simulink model "ROPOD_4Wheel_Tdistkinb_cntr_modular_Code_GEN"  (R2020b)
settings: Solver=VariableStepAuto  StartTime=0.0  StopTime=10.0  RelTol=1e-3
values from neighbouring files (symbols this model uses):
  FFtheta_intia = 0    [init_model.m]
  FFxy_mass = 0*80    (= 0)    [init_model.m]
  I_fhz_dtheta_cntr = 0.3    [init_model.m]
  I_fhz_dvarphi_cntr = 0    [init_model.m]
  I_fhz_dxdy_cntr = 0.25    [init_model.m]
  K_gain_dtheta_cntr = 150    [init_model.m]
  K_gain_dvarphi_cntr = 0.05    [init_model.m]
  K_gain_dxdy_cntr = 200    [init_model.m]
  LL_wp_fhz_dtheta_cntr = 20    [init_model.m]
  LL_wp_fhz_dvarphi_cntr = 10    [init_model.m]
  LL_wp_fhz_dxdy_cntr = 20    [init_model.m]
  LL_wz_fhz_dtheta_cntr = 20    [init_model.m]
  LL_wz_fhz_dvarphi_cntr = 2    [init_model.m]
  LL_wz_fhz_dxdy_cntr = 20    [init_model.m]
  LPF_fhz_ddelta_meas = 50    [init_model.m]
  LPF_fhz_dtheta_cntr = 100    [init_model.m]
  LPF_fhz_dvarphi_cntr = 50    [init_model.m]
  LPF_fhz_dvarphi_meas = 50    [init_model.m]
  LPF_fhz_dxdy_cntr = 100    [init_model.m]
  max_hw_tau = 7.0    (= 7)    [init_model.m]
  max_ropod_acc_theta = 1.6    [init_model.m]
  max_ropod_acc_xy = 2.0    (= 2)    [init_model.m]
  max_ropod_sw_force = 500    [init_model.m]
  max_ropod_sw_tau = 250    [init_model.m]
  max_ropod_vel_theta = 1.6    [init_model.m]
  max_ropod_vel_xy = 2.0    (= 2)    [init_model.m]
  max_sw_current = 10    [init_model.m]
  Nwheels = 4    [Jqwl_numeric_function.m]    (also in S_matrix.m; extract_kinmodel_parameters.m; init_model.m; tau_optimal_dist_vec_fun.m)
  pivot_offs_sws = [0.0243    0.4689    0.3384    5.9050]    [init_model.m]
  ropod_kinmodel_pv = struct2array(ropod_kinmodel_param)    [set_ropod_KinModparams.m]
  SW_COM1_ENABLE1 = hex2dec('0001')    [init_model.m]
  SW_COM1_ENABLE2 = hex2dec('0002')    [init_model.m]
  SW_COM1_MODE_TORQUE = bitshift(hex2dec('0000'),2)    [init_model.m]
  SW_COM1_MODE_VELOCITY = bitshift(hex2dec('0002'),2)    [init_model.m]
  SW_COM1_USE_TS = hex2dec('8000')    [init_model.m]
  sw_tau_2_current = 1/motor_physical_parameters.torqueconstant.value    [init_model.m]
  Tinit = 2    [init_model.m]
  Ts = 0.001    [init_model.m]
undefined symbols (not defined in the file or in its folder): DiscIntNeverNeededParam
libraries: simulink x25, cstblocks x23, pid_lib x22, dspsigops x12, SOEM_EtherCAT_Lib x5
(part 1 of 4)
settings Model: Creator=cesar  LastModifiedBy=cesar
settings DataIOCC: ReturnWorkspaceOutputs=off
settings OptimizationCC: DefaultParameterBehavior=Inlined  UseFloatMulNetSlope=on  InlineInvariantSignals=on  EfficientFloat2IntCast=on
settings DebuggingCC: UnderSpecifiedDataTypeMsg=warning  ArithmeticOperatorsInVariantConditions=warning
settings HardwareCC: ProdBitPerLong=64  ProdHWDeviceType=Intel->x86-64 (Linux 64)
settings SFSimCC: SimUseLocalCustomCode=off  CustomCodeUndefinedFunction=UseInterfaceOnly
settings RTWCC: GenCodeOnly=on  RTWUseLocalCustomCode=off  BuildConfiguration=Faster Runs
settings GRTTargetCC: MatFileLogging=off  SupportNonFinite=off

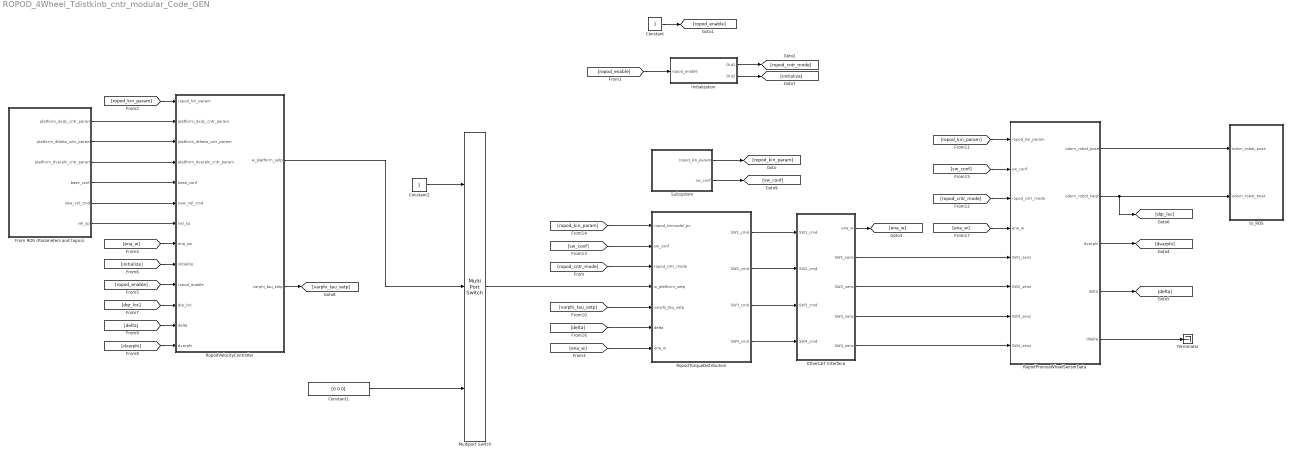
== system ROPOD_4Wheel_Tdistkinb_cntr_modular_Code_GEN ==
  Constant : Constant
  Constant1 : Constant  Value=[0 0 0]
  Constant2 : Constant
  EtherCAT Interface : Subsystem
  From ROS (Parameters and topics) : Subsystem
  Initialization : Subsystem
  Multiport Switch : MultiPortSwitch  Inputs=2
  RopodProcessWheelSensorData : Subsystem
  RopodTorqueDistribution : Subsystem
  RopodVelocityController : Subsystem
  Subsystem : Subsystem
  Terminator : Terminator
  to_ROS : Subsystem
  wires:
  RopodProcessWheelSensorData/1(odom_robot_pose) -> to_ROS/1(odom_robot_pose)
  RopodProcessWheelSensorData/2(odom_robot_twist) -> [dqr_loc], to_ROS/2(odom_robot_twist)
  RopodTorqueDistribution/4(SW4_cmd) -> EtherCAT Interface/4(SW4_cmd)
  RopodTorqueDistribution/3(SW3_cmd) -> EtherCAT Interface/3(SW3_cmd)
  RopodTorqueDistribution/2(SW2_cmd) -> EtherCAT Interface/2(SW2_cmd)
  RopodTorqueDistribution/1(SW1_cmd) -> EtherCAT Interface/1(SW1_cmd)
  From ROS (Parameters and topics)/1(platform_dxdy_cntr_param) -> RopodVelocityController/2(platform_dxdy_cntr_param)
  From ROS (Parameters and topics)/2(platform_dtheta_cntr_param) -> RopodVelocityController/3(platform_dtheta_cntr_param)
  From ROS (Parameters and topics)/3(platform_dvarphi_cntr_param) -> RopodVelocityController/4(platform_dvarphi_cntr_param)
  From ROS (Parameters and topics)/4(base_conf) -> RopodVelocityController/5(base_conf)
  From ROS (Parameters and topics)/5(new_vel_cmd) -> RopodVelocityController/6(new_vel_cmd)
  From ROS (Parameters and topics)/6(vel_sp) -> RopodVelocityController/7(vel_sp)
  [ropod_cntr_mode] -> RopodTorqueDistribution/3(ropod_cntr_mode)
  [ropod_enable] -> Initialization/1(ropod_enable)
  Initialization/1(Out1) -> [ropod_cntr_mode]
  Initialization/2(Out2) -> [initialize]
  Constant/1 -> [ropod_enable]
  [ropod_kin_param] -> RopodVelocityController/1(ropod_kin_param)
  [ena_w] -> RopodTorqueDistribution/7(ena_w)
  [ena_w] -> RopodVelocityController/8(ena_sw)
  [ropod_enable] -> RopodVelocityController/10(ropod_enable)
  [initialize] -> RopodVelocityController/9(initialize)
  RopodProcessWheelSensorData/3(dvarphi) -> [dvarphi]
  RopodProcessWheelSensorData/4(delta) -> [delta]
  RopodProcessWheelSensorData/5(ddelta) -> Terminator/1
  [dqr_loc] -> RopodVelocityController/11(dqr_loc)
  [dvarphi] -> RopodVelocityController/13(dvarphi)
  [delta] -> RopodVelocityController/12(delta)
  RopodVelocityController/2(varphi_tau_setp) -> [varphi_tau_setp]
  [varphi_tau_setp] -> RopodTorqueDistribution/5(varphi_tau_setp)
  Constant2/1 -> Multiport Switch/1
  Constant1/1 -> Multiport Switch/3
  RopodVelocityController/1(w_platform_setp) -> Multiport Switch/2
  [ropod_kin_param] -> RopodProcessWheelSensorData/1(ropod_kin_param)
  [ropod_cntr_mode] -> RopodProcessWheelSensorData/3(ropod_cntr_mode)
  Subsystem/1(ropod_kin_param) -> [ropod_kin_param]
  Subsystem/2(sw_conf) -> [sw_conf]
  [sw_conf] -> RopodTorqueDistribution/2(sw_conf)
  [ropod_kin_param] -> RopodTorqueDistribution/1(ropod_kinmodel_pv)
  [sw_conf] -> RopodProcessWheelSensorData/2(sw_conf)
  EtherCAT Interface/1(ena_w) -> [ena_w]
  EtherCAT Interface/2(SW1_sens) -> RopodProcessWheelSensorData/5(SW1_sens)
  EtherCAT Interface/3(SW2_sens) -> RopodProcessWheelSensorData/6(SW2_sens)
  EtherCAT Interface/4(SW3_sens) -> RopodProcessWheelSensorData/7(SW3_sens)
  EtherCAT Interface/5(SW4_sens) -> RopodProcessWheelSensorData/8(SW4_sens)
  [delta] -> RopodTorqueDistribution/6(delta)
  Multiport Switch/1 -> RopodTorqueDistribution/4(w_platform_setp)
  [ena_w] -> RopodProcessWheelSensorData/4(ena_w)

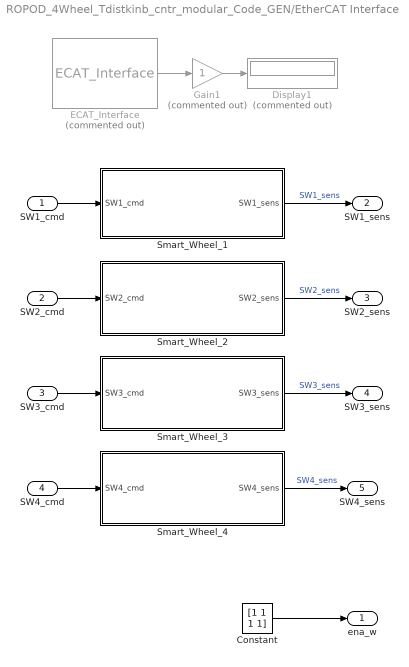
== system ROPOD_4Wheel_Tdistkinb_cntr_modular_Code_GEN/EtherCAT Interface ==
  SW1_cmd : Inport
  SW2_cmd : Inport  Port=2
  SW3_cmd : Inport  Port=3
  SW4_cmd : Inport  Port=4
  Constant : Constant  Value=[1 1 1 1]
  Display1 : Display  Commented=on
  ECAT_Interface : SOEM_EtherCAT_Lib/ECAT_Interface  Priority=0  Commented=on  IFINTERFACE=eth0  TS=Ts
      settings: SourceProductName=SOEM_EtherCAT_Lib
  Gain1 : Gain  Commented=on  OutDataTypeStr=double
  Smart_Wheel_1 : Subsystem
  Smart_Wheel_2 : Subsystem
  Smart_Wheel_3 : Subsystem
  Smart_Wheel_4 : Subsystem
  ena_w : Outport  VectorParamsAs1DForOutWhenUnconnected=off
  SW1_sens : Outport  Port=2  VectorParamsAs1DForOutWhenUnconnected=off
  SW2_sens : Outport  Port=3  VectorParamsAs1DForOutWhenUnconnected=off
  SW3_sens : Outport  Port=4  VectorParamsAs1DForOutWhenUnconnected=off
  SW4_sens : Outport  Port=5  VectorParamsAs1DForOutWhenUnconnected=off
  wires:
  Smart_Wheel_2/1(SW2_sens) -> SW2_sens/1  "SW2_sens"
  Smart_Wheel_3/1(SW3_sens) -> SW3_sens/1  "SW3_sens"
  SW4_cmd/1 -> Smart_Wheel_4/1(SW4_cmd)
  SW2_cmd/1 -> Smart_Wheel_2/1(SW2_cmd)
  SW3_cmd/1 -> Smart_Wheel_3/1(SW3_cmd)
  SW1_cmd/1 -> Smart_Wheel_1/1(SW1_cmd)
  Smart_Wheel_1/1(SW1_sens) -> SW1_sens/1  "SW1_sens"
  Smart_Wheel_4/1(SW4_sens) -> SW4_sens/1  "SW4_sens"
  ECAT_Interface/1 -> Gain1/1
  Gain1/1 -> Display1/1
  Constant/1 -> ena_w/1

== system ROPOD_4Wheel_Tdistkinb_cntr_modular_Code_GEN/From ROS (Parameters and topics) ==
  note: doing the transformation with the angle from odometry data helps
      | to keep the robot better align during the Identification, especially because
      | we do not have any absolute reference
  Constant1 : Constant
  Controllers conf : Subsystem
  From Workspace1 : FromWorkspace  VariableName=qrefdot
  Gain1 : Gain
  ROS base conf : Subsystem
  Selector1 : Selector  InputPortWidth=3  IndexOptions=Index vector (dialog)  Indices=3  OutputSizes=1
  rot_matrix2 : MATLAB Function  TreatAsAtomicUnit=on
  platform_dxdy_cntr_param : Outport  VectorParamsAs1DForOutWhenUnconnected=off
  platform_dtheta_cntr_param : Outport  Port=2  VectorParamsAs1DForOutWhenUnconnected=off
  platform_dvarphi_cntr_param : Outport  Port=3  VectorParamsAs1DForOutWhenUnconnected=off
  base_conf : Outport  Port=4  VectorParamsAs1DForOutWhenUnconnected=off
  new_vel_cmd : Outport  Port=5  VectorParamsAs1DForOutWhenUnconnected=off
  vel_sp : Outport  Port=6  VectorParamsAs1DForOutWhenUnconnected=off
  wires:
  Controllers conf/1(platform_dxdy_cntr_param) -> platform_dxdy_cntr_param/1
  Constant1/1 -> new_vel_cmd/1
  Gain1/1 -> vel_sp/1
  ROS base conf/1(base_conf) -> base_conf/1
  From Workspace1/1 -> Selector1/1, rot_matrix2/1(dqr_glb)
  Controllers conf/3(platform_dvarphi_cntr_param) -> platform_dvarphi_cntr_param/1
  Controllers conf/2(platform_dtheta_cntr_param) -> platform_dtheta_cntr_param/1
  Selector1/1 -> rot_matrix2/2(theta)
  rot_matrix2/1(dqr_loc) -> Gain1/1

== system ROPOD_4Wheel_Tdistkinb_cntr_modular_Code_GEN/Initialization ==
  ropod_enable : Inport
  Allow Tinit seconds for initialization : simulink/Logic and Bit Operations/Compare To Constant  relop=<  const=Tinit  OutDataTypeStr=boolean
  Constant : Constant  Value=2
  Constant1 : Constant
  Constant2 : Constant  Value=0
  Digital Clock : DigitalClock  SampleTime=Ts
  Gain : Gain
  Gain1 : Gain  OutDataTypeStr=double
  Switch : Switch  Criteria=u2 > Threshold
  Switch1 : Switch  Criteria=u2 > Threshold
  Out1 : Outport  VectorParamsAs1DForOutWhenUnconnected=off
  Out2 : Outport  Port=2  VectorParamsAs1DForOutWhenUnconnected=off
  wires:
  Switch/1 -> Switch1/1
  Constant1/1 -> Switch/3
  Switch1/1 -> Gain/1
  Digital Clock/1 -> Allow Tinit seconds for initialization/1
  Allow Tinit seconds for initialization/1 -> Gain1/1, Switch/2
  Constant2/1 -> Switch1/3
  Constant/1 -> Switch/1
  ropod_enable/1 -> Switch1/2
  Gain/1 -> Out1/1
  Gain1/1 -> Out2/1

== system ROPOD_4Wheel_Tdistkinb_cntr_modular_Code_GEN/RopodProcessWheelSensorData ==
  ropod_kin_param : Inport
  sw_conf : Inport  Port=2
  ropod_cntr_mode : Inport  Port=3
  ena_w : Inport  Port=4
  SW1_sens : Inport  Port=5
  SW2_sens : Inport  Port=6
  SW3_sens : Inport  Port=7
  SW4_sens : Inport  Port=8
  Compare To Constant : simulink/Logic and Bit Operations/Compare To Constant  relop=~=  const=1  OutDataTypeStr=boolean
  Odometry and Measurement model 4SW : Subsystem
  ROPOD_4Wheel_sens : Subsystem
  odom_robot_pose : Outport  VectorParamsAs1DForOutWhenUnconnected=off
  odom_robot_twist : Outport  Port=2  VectorParamsAs1DForOutWhenUnconnected=off
  dvarphi : Outport  Port=3  VectorParamsAs1DForOutWhenUnconnected=off
  delta : Outport  Port=4  VectorParamsAs1DForOutWhenUnconnected=off
  ddelta : Outport  Port=5  VectorParamsAs1DForOutWhenUnconnected=off
  wires:
  ropod_kin_param/1 -> Odometry and Measurement model 4SW/1(param_in)
  Odometry and Measurement model 4SW/2(odom_robot_twist) -> odom_robot_twist/1
  SW2_sens/1 -> ROPOD_4Wheel_sens/4(SW2_sens)
  ROPOD_4Wheel_sens/3(ddelta) -> ddelta/1
  Odometry and Measurement model 4SW/1(odom_robot_pose) -> odom_robot_pose/1
  ROPOD_4Wheel_sens/2(delta) -> Odometry and Measurement model 4SW/4(delta), delta/1
  SW4_sens/1 -> ROPOD_4Wheel_sens/6(SW4_sens)
  ROPOD_4Wheel_sens/1(dvarphi) -> Odometry and Measurement model 4SW/3(dvarphi), dvarphi/1
  SW3_sens/1 -> ROPOD_4Wheel_sens/5(SW3_sens)
  SW1_sens/1 -> ROPOD_4Wheel_sens/3(SW1_sens)
  Compare To Constant/1 -> ROPOD_4Wheel_sens/1(disable)
  sw_conf/1 -> ROPOD_4Wheel_sens/2(sw_conf)
  ropod_cntr_mode/1 -> Compare To Constant/1
  ena_w/1 -> Odometry and Measurement model 4SW/2(ena_w)

== system ROPOD_4Wheel_Tdistkinb_cntr_modular_Code_GEN/RopodTorqueDistribution ==
  ropod_kinmodel_pv : Inport
  sw_conf : Inport  Port=2
  ropod_cntr_mode : Inport  Port=3
  w_platform_setp : Inport  Port=4
  varphi_tau_setp : Inport  Port=5
  delta : Inport  Port=6
  ena_w : Inport  Port=7
  Add : Sum
  ROPOD 4SW : Subsystem
  To File1 : ToFile  Filename=varphi_tau_setp.mat  MatrixName=varphi_tau_setp
  Torque distribution : Subsystem
  SW1_cmd : Outport  VectorParamsAs1DForOutWhenUnconnected=off
  SW2_cmd : Outport  Port=2  VectorParamsAs1DForOutWhenUnconnected=off
  SW3_cmd : Outport  Port=3  VectorParamsAs1DForOutWhenUnconnected=off
  SW4_cmd : Outport  Port=4  VectorParamsAs1DForOutWhenUnconnected=off
  wires:
  ROPOD 4SW/4(SW4_cmd) -> SW4_cmd/1
  w_platform_setp/1 -> Torque distribution/1(w_platform_setp)
  ropod_kinmodel_pv/1 -> Torque distribution/2(ropod_kinmodel_pv)
  Add/1 -> ROPOD 4SW/3(varphi_tau_setp), To File1/1
  ROPOD 4SW/1(SW1_cmd) -> SW1_cmd/1
  ena_w/1 -> Torque distribution/5(ena_w)
  ROPOD 4SW/3(SW3_cmd) -> SW3_cmd/1
  ropod_cntr_mode/1 -> ROPOD 4SW/2(ropod_cntr_mode)
  Torque distribution/1(varphi_tau_setp_out) -> Add/2
  [sw_conf] -> ROPOD 4SW/1(sw_conf)
  ROPOD 4SW/2(SW2_cmd) -> SW2_cmd/1
  varphi_tau_setp/1 -> Add/1
  sw_conf/1 -> [sw_conf], Torque distribution/3(sw_conf)
  delta/1 -> Torque distribution/4(delta)

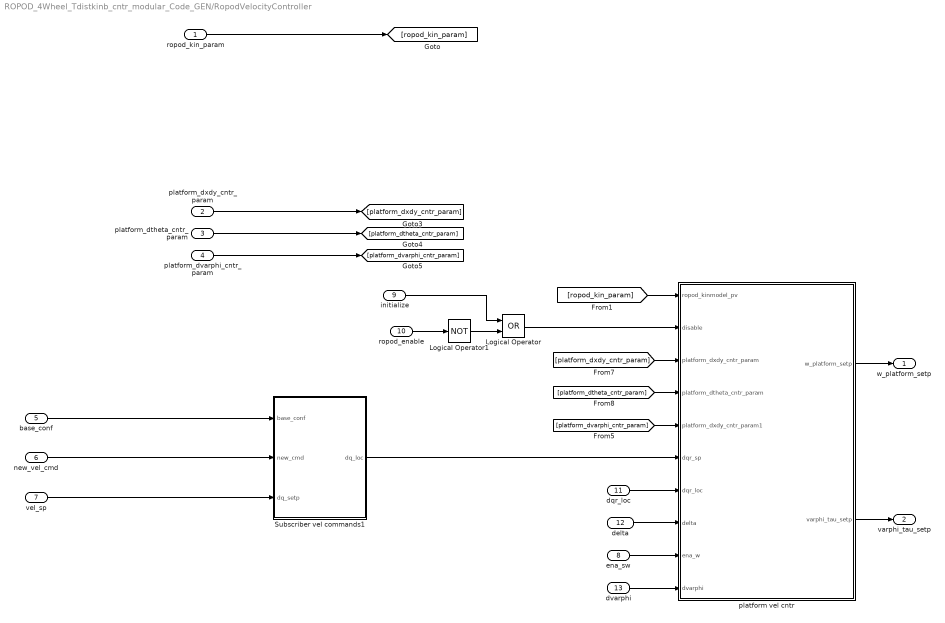
== system ROPOD_4Wheel_Tdistkinb_cntr_modular_Code_GEN/RopodVelocityController ==
  ropod_kin_param : Inport
  platform_dxdy_cntr_param : Inport  Port=2
  platform_dtheta_cntr_param : Inport  Port=3
  platform_dvarphi_cntr_param : Inport  Port=4
  base_conf : Inport  Port=5
  new_vel_cmd : Inport  Port=6
  vel_sp : Inport  Port=7
  ena_sw : Inport  Port=8
  initialize : Inport  Port=9
  ropod_enable : Inport  Port=10
  dqr_loc : Inport  Port=11
  delta : Inport  Port=12
  dvarphi : Inport  Port=13
  Logical Operator : Logic  Operator=OR  AllPortsSameDT=off  OutDataTypeStr=boolean
  Logical Operator1 : Logic  Operator=NOT  AllPortsSameDT=off  OutDataTypeStr=boolean
  Subscriber vel commands1 : Subsystem
  platform vel cntr : Subsystem
  w_platform_setp : Outport  VectorParamsAs1DForOutWhenUnconnected=off
  varphi_tau_setp : Outport  Port=2  VectorParamsAs1DForOutWhenUnconnected=off
  wires:
  platform_dvarphi_cntr_param/1 -> [platform_dvarphi_cntr_param]
  platform_dxdy_cntr_param/1 -> [platform_dxdy_cntr_param]
  ropod_kin_param/1 -> [ropod_kin_param]
  platform_dtheta_cntr_param/1 -> [platform_dtheta_cntr_param]
  [ropod_kin_param] -> platform vel cntr/1(ropod_kinmodel_pv)
  vel_sp/1 -> Subscriber vel commands1/3(dq_setp)
  Subscriber vel commands1/1(dq_loc) -> platform vel cntr/6(dqr_sp)
  base_conf/1 -> Subscriber vel commands1/1(base_conf)
  ena_sw/1 -> platform vel cntr/9(ena_w)
  new_vel_cmd/1 -> Subscriber vel commands1/2(new_cmd)
  [platform_dtheta_cntr_param] -> platform vel cntr/4(platform_dtheta_cntr_param)
  [platform_dxdy_cntr_param] -> platform vel cntr/3(platform_dxdy_cntr_param)
  [platform_dvarphi_cntr_param] -> platform vel cntr/5(platform_dxdy_cntr_param1)
  dqr_loc/1 -> platform vel cntr/7(dqr_loc)
  delta/1 -> platform vel cntr/8(delta)
  dvarphi/1 -> platform vel cntr/10(dvarphi)
  platform vel cntr/2(varphi_tau_setp) -> varphi_tau_setp/1
  platform vel cntr/1(w_platform_setp) -> w_platform_setp/1
  ropod_enable/1 -> Logical Operator1/1
  Logical Operator1/1 -> Logical Operator/2
  Logical Operator/1 -> platform vel cntr/2(disable)
  initialize/1 -> Logical Operator/1

== system ROPOD_4Wheel_Tdistkinb_cntr_modular_Code_GEN/Subsystem ==
  Ropod kinematic parameters : Subsystem
  Smart wheels conf1 : Subsystem
  ropod_kin_param : Outport  VectorParamsAs1DForOutWhenUnconnected=off
  sw_conf : Outport  Port=2  VectorParamsAs1DForOutWhenUnconnected=off
  wires:
  Ropod kinematic parameters/1(ropod_kin_param) -> ropod_kin_param/1
  Smart wheels conf1/1(sw_conf) -> sw_conf/1

== system ROPOD_4Wheel_Tdistkinb_cntr_modular_Code_GEN/to_ROS ==
  odom_robot_pose : Inport
  odom_robot_twist : Inport  Port=2
  Terminator1 : Terminator
  Terminator2 : Terminator
  wires:
  odom_robot_pose/1 -> Terminator2/1
  odom_robot_twist/1 -> Terminator1/1

== system ROPOD_4Wheel_Tdistkinb_cntr_modular_Code_GEN/EtherCAT Interface/Smart_Wheel_1 ==
  SW1_cmd : Inport
  Bus Creator1 : BusCreator  Inputs=40
  Bus Selector : BusSelector  OutputSignals=command1,command2,setpoint1,setpoint2,limit1_p,limit1_n,limit2_p,limit2_n,timestamp
  ec_ROPOD_SmartWheel : SOEM_EtherCAT_Lib/ec_ROPOD_SmartWheel  link_id=1
      settings: SourceProductName=SOEM_EtherCAT_Lib
  SW1_sens : Outport  VectorParamsAs1DForOutWhenUnconnected=off
  wires:
  Bus Creator1/1 -> SW1_sens/1
  ec_ROPOD_SmartWheel/21 -> Bus Creator1/21  "current_2_u"
  ec_ROPOD_SmartWheel/3 -> Bus Creator1/3  "sensor_ts"
  ec_ROPOD_SmartWheel/34 -> Bus Creator1/34  "accel_y"
  ec_ROPOD_SmartWheel/29 -> Bus Creator1/29  "encoder_pivot"
  ec_ROPOD_SmartWheel/18 -> Bus Creator1/18  "velocity_2"
  ec_ROPOD_SmartWheel/19 -> Bus Creator1/19  "current_2_d"
  ec_ROPOD_SmartWheel/14 -> Bus Creator1/14  "voltage_1_v"
  ec_ROPOD_SmartWheel/6 -> Bus Creator1/6  "velocity_1"
  ec_ROPOD_SmartWheel/12 -> Bus Creator1/12  "voltage_1"
  ec_ROPOD_SmartWheel/35 -> Bus Creator1/35  "accel_z"
  ec_ROPOD_SmartWheel/2 -> Bus Creator1/2  "status2"
  ec_ROPOD_SmartWheel/1 -> Bus Creator1/1  "status1"
  ec_ROPOD_SmartWheel/22 -> Bus Creator1/22  "current_2_v"
  ec_ROPOD_SmartWheel/25 -> Bus Creator1/25  "voltage_2_u"
  ec_ROPOD_SmartWheel/24 -> Bus Creator1/24  "voltage_2"
  ec_ROPOD_SmartWheel/15 -> Bus Creator1/15  "voltage_1_w"
  ec_ROPOD_SmartWheel/9 -> Bus Creator1/9  "current_1_u"
  ec_ROPOD_SmartWheel/28 -> Bus Creator1/28  "temperature_2"
  ec_ROPOD_SmartWheel/37 -> Bus Creator1/37  "gyro_y"
  ec_ROPOD_SmartWheel/20 -> Bus Creator1/20  "current_2_q"
  ec_ROPOD_SmartWheel/38 -> Bus Creator1/38  "gyro_z"
  ec_ROPOD_SmartWheel/13 -> Bus Creator1/13  "voltage_1_u"
  ec_ROPOD_SmartWheel/27 -> Bus Creator1/27  "voltage_2_w"
  ec_ROPOD_SmartWheel/7 -> Bus Creator1/7  "current_1_d"
  ec_ROPOD_SmartWheel/5 -> Bus Creator1/5  "encoder_1"
  ec_ROPOD_SmartWheel/36 -> Bus Creator1/36  "gyro_x"
  ec_ROPOD_SmartWheel/23 -> Bus Creator1/23  "current_2_w"
  ec_ROPOD_SmartWheel/4 -> Bus Creator1/4  "setpoint_ts"
  ec_ROPOD_SmartWheel/17 -> Bus Creator1/17  "encoder_2"
  ec_ROPOD_SmartWheel/11 -> Bus Creator1/11  "current_1_w"
  ec_ROPOD_SmartWheel/40 -> Bus Creator1/40  "pressure"
  ec_ROPOD_SmartWheel/30 -> Bus Creator1/30  "velocity_pivot"
  ec_ROPOD_SmartWheel/10 -> Bus Creator1/10  "current_1_v"
  ec_ROPOD_SmartWheel/39 -> Bus Creator1/39  "temperature_imu"
  ec_ROPOD_SmartWheel/16 -> Bus Creator1/16  "temperature_1"
  ec_ROPOD_SmartWheel/33 -> Bus Creator1/33  "accel_x"
  ec_ROPOD_SmartWheel/26 -> Bus Creator1/26  "voltage_2_v"
  ec_ROPOD_SmartWheel/8 -> Bus Creator1/8  "current_1_q"
  ec_ROPOD_SmartWheel/31 -> Bus Creator1/31  "voltage_bus"
  ec_ROPOD_SmartWheel/32 -> Bus Creator1/32  "imu_ts"
  SW1_cmd/1 -> Bus Selector/1
  Bus Selector/1 -> ec_ROPOD_SmartWheel/1  "<command1>"
  Bus Selector/2 -> ec_ROPOD_SmartWheel/2  "<command2>"
  Bus Selector/3 -> ec_ROPOD_SmartWheel/3  "<setpoint1>"
  Bus Selector/4 -> ec_ROPOD_SmartWheel/4  "<setpoint2>"
  Bus Selector/5 -> ec_ROPOD_SmartWheel/5  "<limit1_p>"
  Bus Selector/6 -> ec_ROPOD_SmartWheel/6  "<limit1_n>"
  Bus Selector/7 -> ec_ROPOD_SmartWheel/7  "<limit2_p>"
  Bus Selector/8 -> ec_ROPOD_SmartWheel/8  "<limit2_n>"
  Bus Selector/9 -> ec_ROPOD_SmartWheel/9  "<timestamp>"

== system ROPOD_4Wheel_Tdistkinb_cntr_modular_Code_GEN/EtherCAT Interface/Smart_Wheel_2 ==
  SW2_cmd : Inport
  Bus Creator1 : BusCreator  Inputs=40
  Bus Selector : BusSelector  OutputSignals=command1,command2,setpoint1,setpoint2,limit1_p,limit1_n,limit2_p,limit2_n,timestamp
  ec_ROPOD_SmartWheel : SOEM_EtherCAT_Lib/ec_ROPOD_SmartWheel  link_id=2
      settings: SourceProductName=SOEM_EtherCAT_Lib
  SW2_sens : Outport  VectorParamsAs1DForOutWhenUnconnected=off
  wires:
  Bus Selector/9 -> ec_ROPOD_SmartWheel/9  "<timestamp>"
  Bus Selector/8 -> ec_ROPOD_SmartWheel/8  "<limit2_n>"
  Bus Selector/7 -> ec_ROPOD_SmartWheel/7  "<limit2_p>"
  Bus Selector/6 -> ec_ROPOD_SmartWheel/6  "<limit1_n>"
  Bus Selector/5 -> ec_ROPOD_SmartWheel/5  "<limit1_p>"
  Bus Selector/4 -> ec_ROPOD_SmartWheel/4  "<setpoint2>"
  Bus Selector/3 -> ec_ROPOD_SmartWheel/3  "<setpoint1>"
  Bus Selector/2 -> ec_ROPOD_SmartWheel/2  "<command2>"
  Bus Selector/1 -> ec_ROPOD_SmartWheel/1  "<command1>"
  SW2_cmd/1 -> Bus Selector/1
  ec_ROPOD_SmartWheel/32 -> Bus Creator1/32  "imu_ts"
  ec_ROPOD_SmartWheel/31 -> Bus Creator1/31  "voltage_bus"
  ec_ROPOD_SmartWheel/8 -> Bus Creator1/8  "current_1_q"
  ec_ROPOD_SmartWheel/26 -> Bus Creator1/26  "voltage_2_v"
  ec_ROPOD_SmartWheel/33 -> Bus Creator1/33  "accel_x"
  ec_ROPOD_SmartWheel/16 -> Bus Creator1/16  "temperature_1"
  ec_ROPOD_SmartWheel/39 -> Bus Creator1/39  "temperature_imu"
  ec_ROPOD_SmartWheel/10 -> Bus Creator1/10  "current_1_v"
  ec_ROPOD_SmartWheel/30 -> Bus Creator1/30  "velocity_pivot"
  ec_ROPOD_SmartWheel/40 -> Bus Creator1/40  "pressure"
  ec_ROPOD_SmartWheel/11 -> Bus Creator1/11  "current_1_w"
  ec_ROPOD_SmartWheel/17 -> Bus Creator1/17  "encoder_2"
  ec_ROPOD_SmartWheel/4 -> Bus Creator1/4  "setpoint_ts"
  ec_ROPOD_SmartWheel/23 -> Bus Creator1/23  "current_2_w"
  ec_ROPOD_SmartWheel/36 -> Bus Creator1/36  "gyro_x"
  ec_ROPOD_SmartWheel/5 -> Bus Creator1/5  "encoder_1"
  ec_ROPOD_SmartWheel/7 -> Bus Creator1/7  "current_1_d"
  ec_ROPOD_SmartWheel/27 -> Bus Creator1/27  "voltage_2_w"
  ec_ROPOD_SmartWheel/13 -> Bus Creator1/13  "voltage_1_u"
  ec_ROPOD_SmartWheel/38 -> Bus Creator1/38  "gyro_z"
  ec_ROPOD_SmartWheel/20 -> Bus Creator1/20  "current_2_q"
  ec_ROPOD_SmartWheel/37 -> Bus Creator1/37  "gyro_y"
  ec_ROPOD_SmartWheel/28 -> Bus Creator1/28  "temperature_2"
  ec_ROPOD_SmartWheel/9 -> Bus Creator1/9  "current_1_u"
  ec_ROPOD_SmartWheel/15 -> Bus Creator1/15  "voltage_1_w"
  ec_ROPOD_SmartWheel/24 -> Bus Creator1/24  "voltage_2"
  ec_ROPOD_SmartWheel/25 -> Bus Creator1/25  "voltage_2_u"
  ec_ROPOD_SmartWheel/22 -> Bus Creator1/22  "current_2_v"
  ec_ROPOD_SmartWheel/1 -> Bus Creator1/1  "status1"
  ec_ROPOD_SmartWheel/2 -> Bus Creator1/2  "status2"
  ec_ROPOD_SmartWheel/35 -> Bus Creator1/35  "accel_z"
  ec_ROPOD_SmartWheel/12 -> Bus Creator1/12  "voltage_1"
  ec_ROPOD_SmartWheel/6 -> Bus Creator1/6  "velocity_1"
  ec_ROPOD_SmartWheel/14 -> Bus Creator1/14  "voltage_1_v"
  ec_ROPOD_SmartWheel/19 -> Bus Creator1/19  "current_2_d"
  ec_ROPOD_SmartWheel/18 -> Bus Creator1/18  "velocity_2"
  ec_ROPOD_SmartWheel/29 -> Bus Creator1/29  "encoder_pivot"
  ec_ROPOD_SmartWheel/34 -> Bus Creator1/34  "accel_y"
  ec_ROPOD_SmartWheel/3 -> Bus Creator1/3  "sensor_ts"
  ec_ROPOD_SmartWheel/21 -> Bus Creator1/21  "current_2_u"
  Bus Creator1/1 -> SW2_sens/1

== system ROPOD_4Wheel_Tdistkinb_cntr_modular_Code_GEN/EtherCAT Interface/Smart_Wheel_3 ==
  SW3_cmd : Inport
  Bus Creator1 : BusCreator  Inputs=40
  Bus Selector : BusSelector  OutputSignals=command1,command2,setpoint1,setpoint2,limit1_p,limit1_n,limit2_p,limit2_n,timestamp
  ec_ROPOD_SmartWheel : SOEM_EtherCAT_Lib/ec_ROPOD_SmartWheel  link_id=3
      settings: SourceProductName=SOEM_EtherCAT_Lib
  SW3_sens : Outport  VectorParamsAs1DForOutWhenUnconnected=off
  wires:
  Bus Creator1/1 -> SW3_sens/1
  ec_ROPOD_SmartWheel/21 -> Bus Creator1/21  "current_2_u"
  ec_ROPOD_SmartWheel/3 -> Bus Creator1/3  "sensor_ts"
  ec_ROPOD_SmartWheel/34 -> Bus Creator1/34  "accel_y"
  ec_ROPOD_SmartWheel/29 -> Bus Creator1/29  "encoder_pivot"
  ec_ROPOD_SmartWheel/18 -> Bus Creator1/18  "velocity_2"
  ec_ROPOD_SmartWheel/19 -> Bus Creator1/19  "current_2_d"
  ec_ROPOD_SmartWheel/14 -> Bus Creator1/14  "voltage_1_v"
  ec_ROPOD_SmartWheel/6 -> Bus Creator1/6  "velocity_1"
  ec_ROPOD_SmartWheel/12 -> Bus Creator1/12  "voltage_1"
  ec_ROPOD_SmartWheel/35 -> Bus Creator1/35  "accel_z"
  ec_ROPOD_SmartWheel/2 -> Bus Creator1/2  "status2"
  ec_ROPOD_SmartWheel/1 -> Bus Creator1/1  "status1"
  ec_ROPOD_SmartWheel/22 -> Bus Creator1/22  "current_2_v"
  ec_ROPOD_SmartWheel/25 -> Bus Creator1/25  "voltage_2_u"
  ec_ROPOD_SmartWheel/24 -> Bus Creator1/24  "voltage_2"
  ec_ROPOD_SmartWheel/15 -> Bus Creator1/15  "voltage_1_w"
  ec_ROPOD_SmartWheel/9 -> Bus Creator1/9  "current_1_u"
  ec_ROPOD_SmartWheel/28 -> Bus Creator1/28  "temperature_2"
  ec_ROPOD_SmartWheel/37 -> Bus Creator1/37  "gyro_y"
  ec_ROPOD_SmartWheel/20 -> Bus Creator1/20  "current_2_q"
  ec_ROPOD_SmartWheel/38 -> Bus Creator1/38  "gyro_z"
  ec_ROPOD_SmartWheel/13 -> Bus Creator1/13  "voltage_1_u"
  ec_ROPOD_SmartWheel/27 -> Bus Creator1/27  "voltage_2_w"
  ec_ROPOD_SmartWheel/7 -> Bus Creator1/7  "current_1_d"
  ec_ROPOD_SmartWheel/5 -> Bus Creator1/5  "encoder_1"
  ec_ROPOD_SmartWheel/36 -> Bus Creator1/36  "gyro_x"
  ec_ROPOD_SmartWheel/23 -> Bus Creator1/23  "current_2_w"
  ec_ROPOD_SmartWheel/4 -> Bus Creator1/4  "setpoint_ts"
  ec_ROPOD_SmartWheel/17 -> Bus Creator1/17  "encoder_2"
  ec_ROPOD_SmartWheel/11 -> Bus Creator1/11  "current_1_w"
  ec_ROPOD_SmartWheel/40 -> Bus Creator1/40  "pressure"
  ec_ROPOD_SmartWheel/30 -> Bus Creator1/30  "velocity_pivot"
  ec_ROPOD_SmartWheel/10 -> Bus Creator1/10  "current_1_v"
  ec_ROPOD_SmartWheel/39 -> Bus Creator1/39  "temperature_imu"
  ec_ROPOD_SmartWheel/16 -> Bus Creator1/16  "temperature_1"
  ec_ROPOD_SmartWheel/33 -> Bus Creator1/33  "accel_x"
  ec_ROPOD_SmartWheel/26 -> Bus Creator1/26  "voltage_2_v"
  ec_ROPOD_SmartWheel/8 -> Bus Creator1/8  "current_1_q"
  ec_ROPOD_SmartWheel/31 -> Bus Creator1/31  "voltage_bus"
  ec_ROPOD_SmartWheel/32 -> Bus Creator1/32  "imu_ts"
  SW3_cmd/1 -> Bus Selector/1
  Bus Selector/1 -> ec_ROPOD_SmartWheel/1  "<command1>"
  Bus Selector/2 -> ec_ROPOD_SmartWheel/2  "<command2>"
  Bus Selector/3 -> ec_ROPOD_SmartWheel/3  "<setpoint1>"
  Bus Selector/4 -> ec_ROPOD_SmartWheel/4  "<setpoint2>"
  Bus Selector/5 -> ec_ROPOD_SmartWheel/5  "<limit1_p>"
  Bus Selector/6 -> ec_ROPOD_SmartWheel/6  "<limit1_n>"
  Bus Selector/7 -> ec_ROPOD_SmartWheel/7  "<limit2_p>"
  Bus Selector/8 -> ec_ROPOD_SmartWheel/8  "<limit2_n>"
  Bus Selector/9 -> ec_ROPOD_SmartWheel/9  "<timestamp>"

== system ROPOD_4Wheel_Tdistkinb_cntr_modular_Code_GEN/EtherCAT Interface/Smart_Wheel_4 ==
  SW4_cmd : Inport
  Bus Creator1 : BusCreator  Inputs=40
  Bus Selector : BusSelector  OutputSignals=command1,command2,setpoint1,setpoint2,limit1_p,limit1_n,limit2_p,limit2_n,timestamp
  ec_ROPOD_SmartWheel : SOEM_EtherCAT_Lib/ec_ROPOD_SmartWheel  link_id=4
      settings: SourceProductName=SOEM_EtherCAT_Lib
  SW4_sens : Outport  VectorParamsAs1DForOutWhenUnconnected=off
  wires:
  Bus Selector/9 -> ec_ROPOD_SmartWheel/9  "<timestamp>"
  Bus Selector/8 -> ec_ROPOD_SmartWheel/8  "<limit2_n>"
  Bus Selector/7 -> ec_ROPOD_SmartWheel/7  "<limit2_p>"
  Bus Selector/6 -> ec_ROPOD_SmartWheel/6  "<limit1_n>"
  Bus Selector/5 -> ec_ROPOD_SmartWheel/5  "<limit1_p>"
  Bus Selector/4 -> ec_ROPOD_SmartWheel/4  "<setpoint2>"
  Bus Selector/3 -> ec_ROPOD_SmartWheel/3  "<setpoint1>"
  Bus Selector/2 -> ec_ROPOD_SmartWheel/2  "<command2>"
  Bus Selector/1 -> ec_ROPOD_SmartWheel/1  "<command1>"
  SW4_cmd/1 -> Bus Selector/1
  ec_ROPOD_SmartWheel/32 -> Bus Creator1/32  "imu_ts"
  ec_ROPOD_SmartWheel/31 -> Bus Creator1/31  "voltage_bus"
  ec_ROPOD_SmartWheel/8 -> Bus Creator1/8  "current_1_q"
  ec_ROPOD_SmartWheel/26 -> Bus Creator1/26  "voltage_2_v"
  ec_ROPOD_SmartWheel/33 -> Bus Creator1/33  "accel_x"
  ec_ROPOD_SmartWheel/16 -> Bus Creator1/16  "temperature_1"
  ec_ROPOD_SmartWheel/39 -> Bus Creator1/39  "temperature_imu"
  ec_ROPOD_SmartWheel/10 -> Bus Creator1/10  "current_1_v"
  ec_ROPOD_SmartWheel/30 -> Bus Creator1/30  "velocity_pivot"
  ec_ROPOD_SmartWheel/40 -> Bus Creator1/40  "pressure"
  ec_ROPOD_SmartWheel/11 -> Bus Creator1/11  "current_1_w"
  ec_ROPOD_SmartWheel/17 -> Bus Creator1/17  "encoder_2"
  ec_ROPOD_SmartWheel/4 -> Bus Creator1/4  "setpoint_ts"
  ec_ROPOD_SmartWheel/23 -> Bus Creator1/23  "current_2_w"
  ec_ROPOD_SmartWheel/36 -> Bus Creator1/36  "gyro_x"
  ec_ROPOD_SmartWheel/5 -> Bus Creator1/5  "encoder_1"
  ec_ROPOD_SmartWheel/7 -> Bus Creator1/7  "current_1_d"
  ec_ROPOD_SmartWheel/27 -> Bus Creator1/27  "voltage_2_w"
  ec_ROPOD_SmartWheel/13 -> Bus Creator1/13  "voltage_1_u"
  ec_ROPOD_SmartWheel/38 -> Bus Creator1/38  "gyro_z"
  ec_ROPOD_SmartWheel/20 -> Bus Creator1/20  "current_2_q"
  ec_ROPOD_SmartWheel/37 -> Bus Creator1/37  "gyro_y"
  ec_ROPOD_SmartWheel/28 -> Bus Creator1/28  "temperature_2"
  ec_ROPOD_SmartWheel/9 -> Bus Creator1/9  "current_1_u"
  ec_ROPOD_SmartWheel/15 -> Bus Creator1/15  "voltage_1_w"
  ec_ROPOD_SmartWheel/24 -> Bus Creator1/24  "voltage_2"
  ec_ROPOD_SmartWheel/25 -> Bus Creator1/25  "voltage_2_u"
  ec_ROPOD_SmartWheel/22 -> Bus Creator1/22  "current_2_v"
  ec_ROPOD_SmartWheel/1 -> Bus Creator1/1  "status1"
  ec_ROPOD_SmartWheel/2 -> Bus Creator1/2  "status2"
  ec_ROPOD_SmartWheel/35 -> Bus Creator1/35  "accel_z"
  ec_ROPOD_SmartWheel/12 -> Bus Creator1/12  "voltage_1"
  ec_ROPOD_SmartWheel/6 -> Bus Creator1/6  "velocity_1"
  ec_ROPOD_SmartWheel/14 -> Bus Creator1/14  "voltage_1_v"
  ec_ROPOD_SmartWheel/19 -> Bus Creator1/19  "current_2_d"
  ec_ROPOD_SmartWheel/18 -> Bus Creator1/18  "velocity_2"
  ec_ROPOD_SmartWheel/29 -> Bus Creator1/29  "encoder_pivot"
  ec_ROPOD_SmartWheel/34 -> Bus Creator1/34  "accel_y"
  ec_ROPOD_SmartWheel/3 -> Bus Creator1/3  "sensor_ts"
  ec_ROPOD_SmartWheel/21 -> Bus Creator1/21  "current_2_u"
  Bus Creator1/1 -> SW4_sens/1

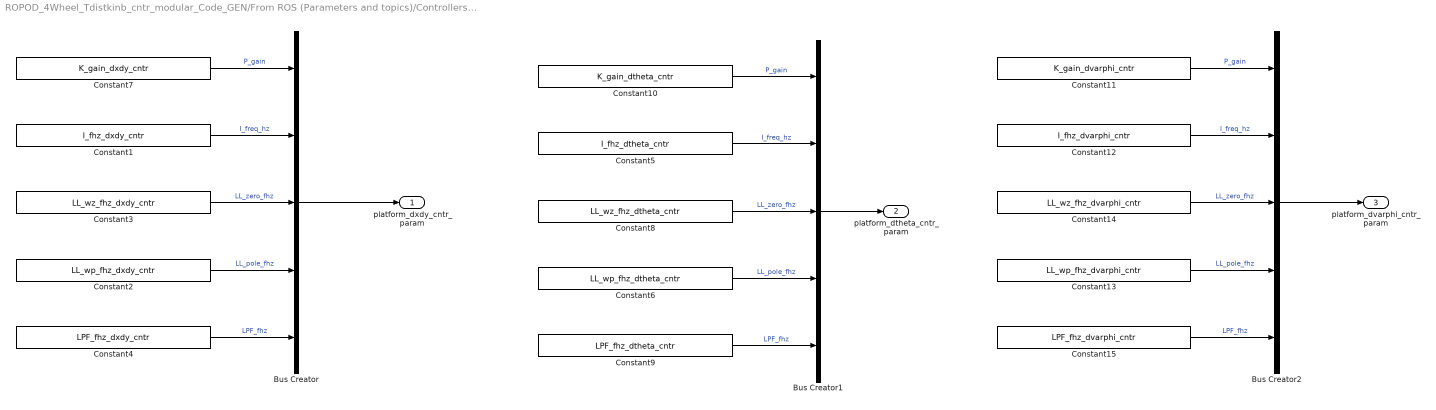
== system ROPOD_4Wheel_Tdistkinb_cntr_modular_Code_GEN/From ROS (Parameters and topics)/Controllers conf ==
  Bus Creator : BusCreator  Inputs=5
  Bus Creator1 : BusCreator  Inputs=5
  Bus Creator2 : BusCreator  Inputs=5
  Constant1 : Constant  Value=I_fhz_dxdy_cntr
  Constant10 : Constant  Value=K_gain_dtheta_cntr
  Constant11 : Constant  Value=K_gain_dvarphi_cntr
  Constant12 : Constant  Value=I_fhz_dvarphi_cntr
  Constant13 : Constant  Value=LL_wp_fhz_dvarphi_cntr
  Constant14 : Constant  Value=LL_wz_fhz_dvarphi_cntr
  Constant15 : Constant  Value=LPF_fhz_dvarphi_cntr
  Constant2 : Constant  Value=LL_wp_fhz_dxdy_cntr
  Constant3 : Constant  Value=LL_wz_fhz_dxdy_cntr
  Constant4 : Constant  Value=LPF_fhz_dxdy_cntr
  Constant5 : Constant  Value=I_fhz_dtheta_cntr
  Constant6 : Constant  Value=LL_wp_fhz_dtheta_cntr
  Constant7 : Constant  Value=K_gain_dxdy_cntr
  Constant8 : Constant  Value=LL_wz_fhz_dtheta_cntr
  Constant9 : Constant  Value=LPF_fhz_dtheta_cntr
  platform_dxdy_cntr_param : Outport  VectorParamsAs1DForOutWhenUnconnected=off
  platform_dtheta_cntr_param : Outport  Port=2  VectorParamsAs1DForOutWhenUnconnected=off
  platform_dvarphi_cntr_param : Outport  Port=3  VectorParamsAs1DForOutWhenUnconnected=off
  wires:
  Constant2/1 -> Bus Creator/4  "LL_pole_fhz"
  Constant4/1 -> Bus Creator/5  "LPF_fhz"
  Bus Creator/1 -> platform_dxdy_cntr_param/1
  Constant1/1 -> Bus Creator/2  "I_freq_hz"
  Constant3/1 -> Bus Creator/3  "LL_zero_fhz"
  Constant7/1 -> Bus Creator/1  "P_gain"
  Bus Creator1/1 -> platform_dtheta_cntr_param/1
  Bus Creator2/1 -> platform_dvarphi_cntr_param/1
  Constant5/1 -> Bus Creator1/2  "I_freq_hz"
  Constant6/1 -> Bus Creator1/4  "LL_pole_fhz"
  Constant10/1 -> Bus Creator1/1  "P_gain"
  Constant8/1 -> Bus Creator1/3  "LL_zero_fhz"
  Constant9/1 -> Bus Creator1/5  "LPF_fhz"
  Constant15/1 -> Bus Creator2/5  "LPF_fhz"
  Constant12/1 -> Bus Creator2/2  "I_freq_hz"
  Constant14/1 -> Bus Creator2/3  "LL_zero_fhz"
  Constant11/1 -> Bus Creator2/1  "P_gain"
  Constant13/1 -> Bus Creator2/4  "LL_pole_fhz"

== system ROPOD_4Wheel_Tdistkinb_cntr_modular_Code_GEN/From ROS (Parameters and topics)/ROS base conf ==
  Bus Creator : BusCreator  Inputs=4
  max_ropod_acc_theta : Constant  Value=max_ropod_acc_theta
  max_ropod_acc_xy : Constant  Value=max_ropod_acc_xy
  max_ropod_vel_theta : Constant  Value=max_ropod_vel_theta
  max_ropod_vel_xy : Constant  Value=max_ropod_vel_xy
  base_conf : Outport  VectorParamsAs1DForOutWhenUnconnected=off
  wires:
  max_ropod_acc_xy/1 -> Bus Creator/2  "max_acc_xy"
  max_ropod_vel_xy/1 -> Bus Creator/1  "max_vel_xy"
  Bus Creator/1 -> base_conf/1
  max_ropod_acc_theta/1 -> Bus Creator/4  "max_acc_theta"
  max_ropod_vel_theta/1 -> Bus Creator/3  "max_vel_theta"

== system ROPOD_4Wheel_Tdistkinb_cntr_modular_Code_GEN/RopodProcessWheelSensorData/Odometry and Measurement model 4SW ==
  note: This output is only useful when using ros
      | This data is fed to /odom/pose
  note: This part is in global coordinates
  note: This part is in local coordinates
  param_in : Inport
  ena_w : Inport  Port=2
  dvarphi : Inport  Port=3
  delta : Inport  Port=4
  Discrete-Time Integrator : DiscreteIntegrator  SampleTime=Ts  ICPrevOutput=DiscIntNeverNeededParam  ICPrevScaledInput=DiscIntNeverNeededParam
  Jqwl_numeric : MATLAB Function  TreatAsAtomicUnit=on
  Selector3 : Selector  InputPortWidth=3  IndexOptions=Index vector (dialog)  Indices=3  OutputSizes=1
  Signal Specification : SignalSpecification  Dimensions=[3 1]
  pos_rot_matrix : MATLAB Function  TreatAsAtomicUnit=on
  odom_robot_pose : Outport  VectorParamsAs1DForOutWhenUnconnected=off
  odom_robot_twist : Outport  Port=2  VectorParamsAs1DForOutWhenUnconnected=off
  wires:
  Jqwl_numeric/1(v) -> Signal Specification/1
  param_in/1 -> Jqwl_numeric/1(ropod_kinmodel_param_vec)
  delta/1 -> Jqwl_numeric/2(delta)
  Signal Specification/1 -> pos_rot_matrix/1(dqr_loc), odom_robot_twist/1
  Selector3/1 -> pos_rot_matrix/2(theta_odom)
  pos_rot_matrix/1(dqr_glb) -> Discrete-Time Integrator/1
  Discrete-Time Integrator/1 -> odom_robot_pose/1, Selector3/1
  dvarphi/1 -> Jqwl_numeric/3(dvarphi)
  ena_w/1 -> Jqwl_numeric/4(ena_w)

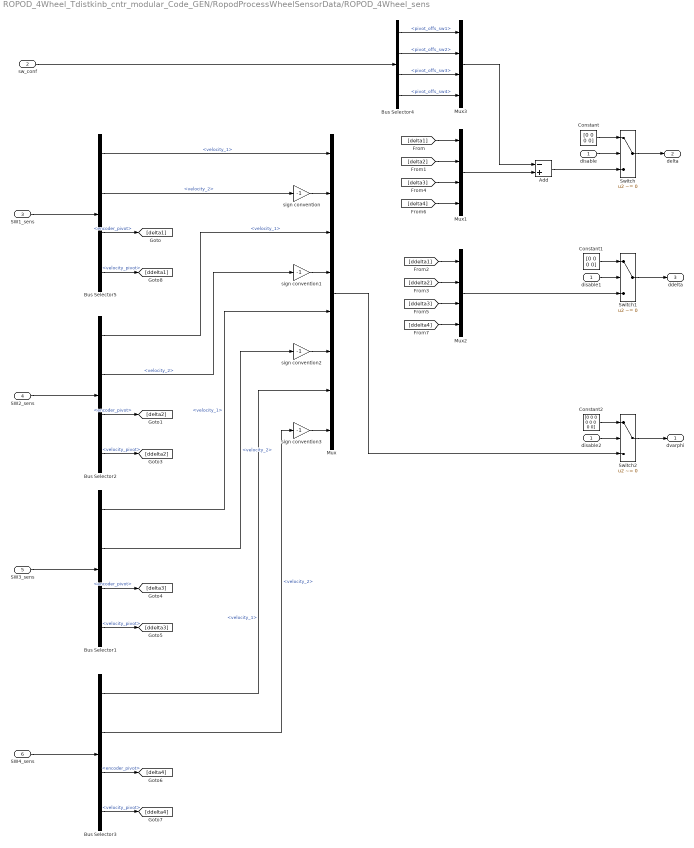
== system ROPOD_4Wheel_Tdistkinb_cntr_modular_Code_GEN/RopodProcessWheelSensorData/ROPOD_4Wheel_sens ==
  disable : Inport
  sw_conf : Inport  Port=2
  SW1_sens : Inport  Port=3
  SW2_sens : Inport  Port=4
  SW3_sens : Inport  Port=5
  SW4_sens : Inport  Port=6
  Add : Sum  Inputs=-+
  Bus Selector{1..3,5} (4 alike) : BusSelector  OutputSignals=velocity_1,velocity_2,encoder_pivot,velocity_pivot
  Bus Selector4 : BusSelector  OutputSignals=pivot_offs_sw1,pivot_offs_sw2,pivot_offs_sw3,pivot_offs_sw4
  Constant : Constant  Value=[0 0 0 0]
  Constant1 : Constant  Value=[0 0 0 0]
  Constant2 : Constant  Value=[0 0 0 0 0 0 0 0]
  Mux : Mux  Inputs=8
  Mux1 : Mux
  Mux2 : Mux
  Mux3 : Mux
  Switch : Switch  Criteria=u2 ~= 0
  Switch1 : Switch  Criteria=u2 ~= 0
  Switch2 : Switch  Criteria=u2 ~= 0
  disable1 : InportShadow
  disable2 : InportShadow
  sign convention{,1..3} (4 alike) : Gain  Gain=-1
  dvarphi : Outport  VectorParamsAs1DForOutWhenUnconnected=off
  delta : Outport  Port=2  VectorParamsAs1DForOutWhenUnconnected=off
  ddelta : Outport  Port=3  VectorParamsAs1DForOutWhenUnconnected=off
  wires:
  SW1_sens/1 -> Bus Selector5/1
  SW2_sens/1 -> Bus Selector2/1
  Bus Selector5/1 -> Mux/1  "<velocity_1>"
  Bus Selector5/2 -> sign convention/1  "<velocity_2>"
  Bus Selector2/1 -> Mux/3  "<velocity_1>"
  Bus Selector2/2 -> sign convention1/1  "<velocity_2>"
  Bus Selector2/3 -> [delta2]  "<encoder_pivot>"
  [delta1] -> Mux1/1
  [delta2] -> Mux1/2
  Bus Selector2/4 -> [ddelta2]  "<velocity_pivot>"
  [ddelta2] -> Mux2/2
  [ddelta1] -> Mux2/1
  Bus Selector1/4 -> [ddelta3]  "<velocity_pivot>"
  Bus Selector1/3 -> [delta3]  "<encoder_pivot>"
  Bus Selector1/2 -> sign convention2/1  "<velocity_2>"
  Bus Selector1/1 -> Mux/5  "<velocity_1>"
  SW3_sens/1 -> Bus Selector1/1
  [delta3] -> Mux1/3
  [ddelta3] -> Mux2/3
  SW4_sens/1 -> Bus Selector3/1
  Bus Selector3/1 -> Mux/7  "<velocity_1>"
  Bus Selector3/2 -> sign convention3/1  "<velocity_2>"
  Bus Selector3/3 -> [delta4]  "<encoder_pivot>"
  Bus Selector3/4 -> [ddelta4]  "<velocity_pivot>"
  [delta4] -> Mux1/4
  [ddelta4] -> Mux2/4
  Mux1/1 -> Add/2
  Mux3/1 -> Add/1
  sw_conf/1 -> Bus Selector4/1
  Bus Selector4/1 -> Mux3/1  "<pivot_offs_sw1>"
  Bus Selector4/2 -> Mux3/2  "<pivot_offs_sw2>"
  Bus Selector4/3 -> Mux3/3  "<pivot_offs_sw3>"
  Bus Selector4/4 -> Mux3/4  "<pivot_offs_sw4>"
  Bus Selector5/3 -> [delta1]  "<encoder_pivot>"
  Bus Selector5/4 -> [ddelta1]  "<velocity_pivot>"
  sign convention/1 -> Mux/2
  sign convention1/1 -> Mux/4
  sign convention2/1 -> Mux/6
  sign convention3/1 -> Mux/8
  Add/1 -> Switch/3
  Switch/1 -> delta/1
  disable/1 -> Switch/2
  Constant/1 -> Switch/1
  Switch1/1 -> ddelta/1
  Mux2/1 -> Switch1/3
  Constant1/1 -> Switch1/1
  disable1/1 -> Switch1/2
  disable2/1 -> Switch2/2
  Constant2/1 -> Switch2/1
  Mux/1 -> Switch2/3
  Switch2/1 -> dvarphi/1

== system ROPOD_4Wheel_Tdistkinb_cntr_modular_Code_GEN/RopodTorqueDistribution/ROPOD 4SW ==
  note: disable = 0, current = 1, initialize = 2
  sw_conf : Inport
  ropod_cntr_mode : Inport  Port=2
  varphi_tau_setp : Inport  Port=3
  Bus Creator : BusCreator  Commented=on  Inputs=4
  Bus Creator1 : BusCreator  Commented=on  Inputs=4
  Gain3 : Gain  Gain=sw_tau_2_current
  Initialization switch : Subsystem
  ROPOD_4Wheel_sens_own_vel_filter : Subsystem  Commented=on
  ROPOD_4Wheel_torque_cmd : Subsystem
  To File : ToFile  Commented=on  Filename=all_wheel_out_data  MatrixName=all_wheel_out_data
  To File2 : ToFile  Commented=on  Filename=all_wheel_in_data  MatrixName=all_wheel_in_data
  empywheel : Subsystem  Commented=on
  SW1_cmd : Outport  VectorParamsAs1DForOutWhenUnconnected=off
  SW2_cmd : Outport  Port=2  VectorParamsAs1DForOutWhenUnconnected=off
  SW3_cmd : Outport  Port=3  VectorParamsAs1DForOutWhenUnconnected=off
  SW4_cmd : Outport  Port=4  VectorParamsAs1DForOutWhenUnconnected=off
  wires:
  ROPOD_4Wheel_torque_cmd/4(SW4_cmd) -> SW4_cmd/1, Bus Creator1/4  "SW4_cmd"
  ROPOD_4Wheel_torque_cmd/1(SW1_cmd) -> SW1_cmd/1, Bus Creator1/1  "SW1_cmd"
  ROPOD_4Wheel_torque_cmd/3(SW3_cmd) -> SW3_cmd/1, Bus Creator1/3  "SW3_cmd"
  sw_conf/1 -> ROPOD_4Wheel_torque_cmd/1(sw_conf)
  ROPOD_4Wheel_torque_cmd/2(SW2_cmd) -> SW2_cmd/1, Bus Creator1/2  "SW2_cmd"
  Bus Creator/1 -> To File/1
  Bus Creator1/1 -> To File2/1
  varphi_tau_setp/1 -> Gain3/1
  Gain3/1 -> Initialization switch/2(curr_setp)
  ropod_cntr_mode/1 -> Initialization switch/1(ropod_cntr_mode)
  Initialization switch/1(SW_cntr_mode) -> ROPOD_4Wheel_torque_cmd/2(cntr_mode)
  Initialization switch/2(wheel_setp) -> ROPOD_4Wheel_torque_cmd/3(wheel_setp)

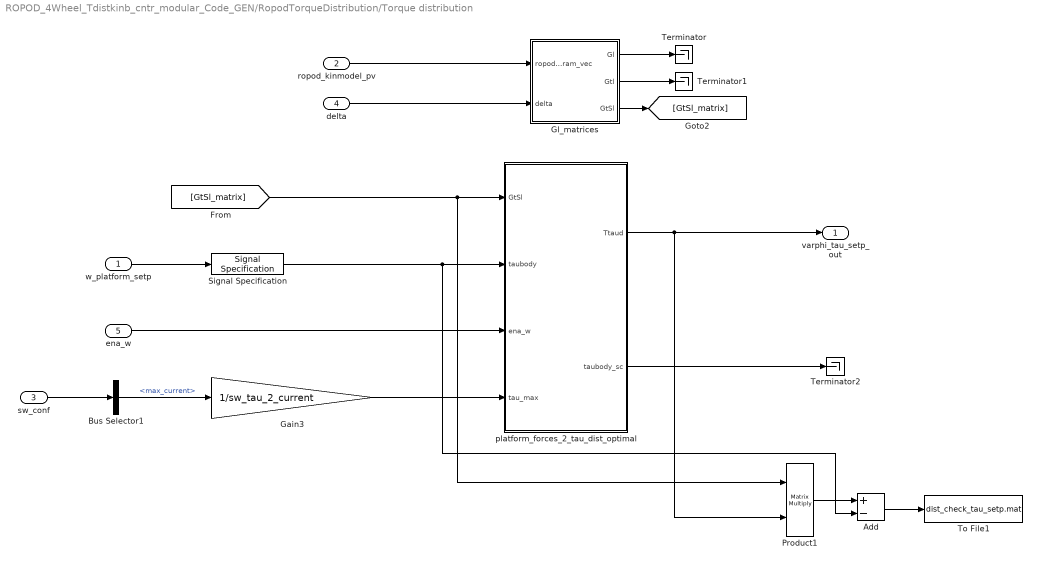
== system ROPOD_4Wheel_Tdistkinb_cntr_modular_Code_GEN/RopodTorqueDistribution/Torque distribution ==
  w_platform_setp : Inport
  ropod_kinmodel_pv : Inport  Port=2
  sw_conf : Inport  Port=3
  delta : Inport  Port=4
  ena_w : Inport  Port=5
  Add : Sum  Inputs=+-
  Bus Selector1 : BusSelector  OutputSignals=max_current
  Gain3 : Gain  Gain=1/sw_tau_2_current
  Gl_matrices : MATLAB Function  TreatAsAtomicUnit=on
  Product1 : Product  Multiplication=Matrix(*)
  Signal Specification : SignalSpecification  Dimensions=[3 1]
  Terminator : Terminator
  Terminator1 : Terminator
  Terminator2 : Terminator
  To File1 : ToFile  Filename=dist_check_tau_setp.mat  MatrixName=dist_check_tau_setp
  platform_forces_2_tau_dist_optimal : MATLAB Function  TreatAsAtomicUnit=on
  varphi_tau_setp_out : Outport  VectorParamsAs1DForOutWhenUnconnected=off
  wires:
  Gl_matrices/3(GtSl) -> [GtSl_matrix]
  Gl_matrices/1(Gl) -> Terminator/1
  delta/1 -> Gl_matrices/2(delta)
  Gl_matrices/2(Gtl) -> Terminator1/1
  ropod_kinmodel_pv/1 -> Gl_matrices/1(ropod_kinmodel_param_vec)
  Bus Selector1/1 -> Gain3/1  "<max_current>"
  sw_conf/1 -> Bus Selector1/1
  Gain3/1 -> platform_forces_2_tau_dist_optimal/4(tau_max)
  ena_w/1 -> platform_forces_2_tau_dist_optimal/3(ena_w)
  [GtSl_matrix] -> platform_forces_2_tau_dist_optimal/1(GtSl), Product1/1
  w_platform_setp/1 -> Signal Specification/1
  platform_forces_2_tau_dist_optimal/2(taubody_sc) -> Terminator2/1
  platform_forces_2_tau_dist_optimal/1(Ttaud) -> Product1/2, varphi_tau_setp_out/1
  Product1/1 -> Add/1
  Add/1 -> To File1/1
  Signal Specification/1 -> platform_forces_2_tau_dist_optimal/2(taubody), Add/2

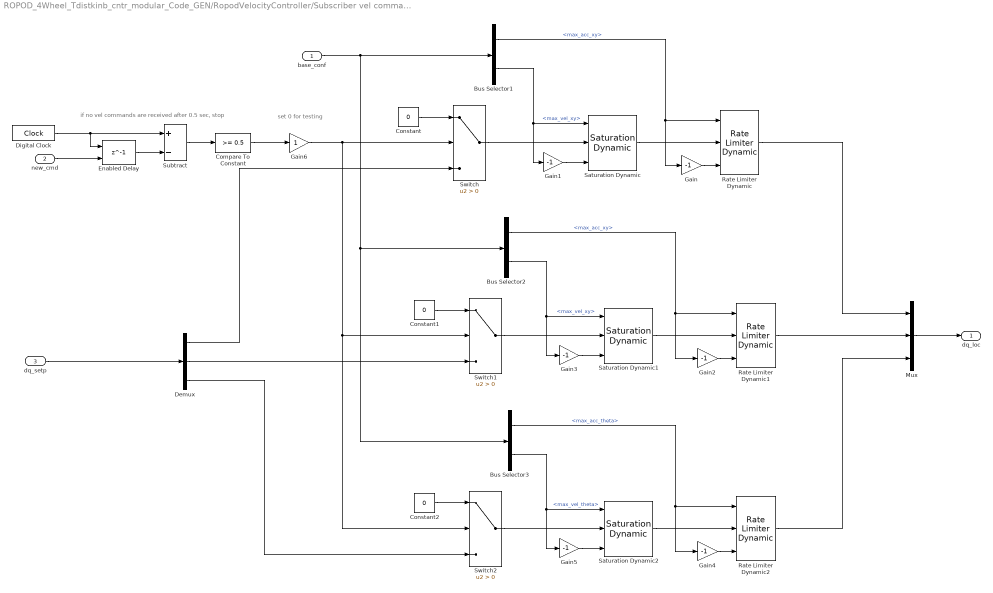
== system ROPOD_4Wheel_Tdistkinb_cntr_modular_Code_GEN/RopodVelocityController/Subscriber vel commands1 ==
  note: set 0 for testing
  note: if no vel commands are received after 0.5 sec, stop
  base_conf : Inport
  new_cmd : Inport  Port=2
  dq_setp : Inport  Port=3
  Bus Selector1 : BusSelector  OutputSignals=max_acc_xy,max_vel_xy
  Bus Selector2 : BusSelector  OutputSignals=max_acc_xy,max_vel_xy
  Bus Selector3 : BusSelector  OutputSignals=max_acc_theta,max_vel_theta
  Compare To Constant : simulink/Logic and Bit Operations/Compare To Constant  relop=>=  const=0.5  OutDataTypeStr=boolean
  Constant : Constant  Value=0  SampleTime=Ts
  Constant1 : Constant  Value=0
  Constant2 : Constant  Value=0
  Demux : Demux  Outputs=3
  Digital Clock : DigitalClock  SampleTime=Ts
  Enabled Delay : Delay  DelayLength=1  ShowEnablePort=on  SampleTime=Ts
      settings: InputPortMap=u0,e6
  Gain{,1..5} (6 alike) : Gain  Gain=-1
  Gain6 : Gain
  Mux : Mux  Inputs=3
  Rate Limiter Dynamic : simulink/Discontinuities/Rate Limiter Dynamic
  Rate Limiter Dynamic1 : simulink/Discontinuities/Rate Limiter Dynamic
  Rate Limiter Dynamic2 : simulink/Discontinuities/Rate Limiter Dynamic
  Saturation Dynamic : simulink/Discontinuities/Saturation Dynamic  OutMin=[]  OutMax=[]  OutDataTypeStr=Inherit: Same as second input  OutDataType=fixdt(1, 16)  OutScaling=2^-10  DoSatur=off
  Saturation Dynamic1 : simulink/Discontinuities/Saturation Dynamic  OutMin=[]  OutMax=[]  OutDataTypeStr=Inherit: Same as second input  OutDataType=fixdt(1, 16)  OutScaling=2^-10  DoSatur=off
  Saturation Dynamic2 : simulink/Discontinuities/Saturation Dynamic  OutMin=[]  OutMax=[]  OutDataTypeStr=Inherit: Same as second input  OutDataType=fixdt(1, 16)  OutScaling=2^-10  DoSatur=off
  Subtract : Sum  Inputs=+-
  Switch : Switch  Criteria=u2 > Threshold
  Switch1 : Switch  Criteria=u2 > Threshold
  Switch2 : Switch  Criteria=u2 > Threshold
  dq_loc : Outport  VectorParamsAs1DForOutWhenUnconnected=off
  wires:
  Demux/1 -> Switch/3
  dq_setp/1 -> Demux/1
  new_cmd/1 -> Enabled Delay/2
  Digital Clock/1 -> Enabled Delay/1, Subtract/1
  Enabled Delay/1 -> Subtract/2
  Subtract/1 -> Compare To Constant/1
  Constant/1 -> Switch/1
  Gain/1 -> Rate Limiter Dynamic/3
  Switch/1 -> Saturation Dynamic/2
  Gain1/1 -> Saturation Dynamic/3
  Saturation Dynamic/1 -> Rate Limiter Dynamic/2
  Switch1/1 -> Saturation Dynamic1/2
  Gain3/1 -> Saturation Dynamic1/3
  Constant1/1 -> Switch1/1
  Demux/2 -> Switch1/3
  Gain2/1 -> Rate Limiter Dynamic1/3
  Saturation Dynamic1/1 -> Rate Limiter Dynamic1/2
  Bus Selector2/1 -> Rate Limiter Dynamic1/1, Gain2/1  "<max_acc_xy>"
  Bus Selector2/2 -> Saturation Dynamic1/1, Gain3/1  "<max_vel_xy>"
  Bus Selector3/1 -> Rate Limiter Dynamic2/1, Gain4/1  "<max_acc_theta>"
  Saturation Dynamic2/1 -> Rate Limiter Dynamic2/2
  base_conf/1 -> Bus Selector3/1, Bus Selector2/1, Bus Selector1/1
  Switch2/1 -> Saturation Dynamic2/2
  Constant2/1 -> Switch2/1
  Demux/3 -> Switch2/3
  Gain5/1 -> Saturation Dynamic2/3
  Gain4/1 -> Rate Limiter Dynamic2/3
  Compare To Constant/1 -> Gain6/1
  Bus Selector3/2 -> Saturation Dynamic2/1, Gain5/1  "<max_vel_theta>"
  Mux/1 -> dq_loc/1
  Rate Limiter Dynamic/1 -> Mux/1
  Rate Limiter Dynamic1/1 -> Mux/2
  Rate Limiter Dynamic2/1 -> Mux/3
  Bus Selector1/2 -> Saturation Dynamic/1, Gain1/1  "<max_vel_xy>"
  Bus Selector1/1 -> Rate Limiter Dynamic/1, Gain/1  "<max_acc_xy>"
  Gain6/1 -> Switch2/2, Switch1/2, Switch/2

== system ROPOD_4Wheel_Tdistkinb_cntr_modular_Code_GEN/RopodVelocityController/platform vel cntr ==
  ropod_kinmodel_pv : Inport
  disable : Inport  Port=2
  platform_dxdy_cntr_param : Inport  Port=3
  platform_dtheta_cntr_param : Inport  Port=4
  platform_dxdy_cntr_param1 : Inport  Port=5
  dqr_sp : Inport  Port=6
  dqr_loc : Inport  Port=7
  delta : Inport  Port=8
  ena_w : Inport  Port=9
  dvarphi : Inport  Port=10
  Inverse Kinematics 4SW : Subsystem
  Platorm Velocity controller : Subsystem
  disable1 : InportShadow  Port=2
  wheel vel cntr : Subsystem
  w_platform_setp : Outport  VectorParamsAs1DForOutWhenUnconnected=off
  varphi_tau_setp : Outport  Port=2  VectorParamsAs1DForOutWhenUnconnected=off
  wires:
  delta/1 -> Inverse Kinematics 4SW/3(delta)
  ropod_kinmodel_pv/1 -> Inverse Kinematics 4SW/1(param_in)
  Platorm Velocity controller/1(w_platform_setp) -> w_platform_setp/1
  disable/1 -> Platorm Velocity controller/1(reset_int)
  dqr_sp/1 -> Platorm Velocity controller/2(dqr_sp), Inverse Kinematics 4SW/2(dqr_sp)
  dqr_loc/1 -> Platorm Velocity controller/3(dqr_loc)
  platform_dxdy_cntr_param/1 -> Platorm Velocity controller/4(platform_dxdy_cntr_param)
  platform_dtheta_cntr_param/1 -> Platorm Velocity controller/5(platform_dtheta_cntr_param)
  Inverse Kinematics 4SW/1(wheel_vel_sp) -> wheel vel cntr/3(dvarphi_sp)
  wheel vel cntr/1(varphi_tau_setp_out) -> varphi_tau_setp/1
  platform_dxdy_cntr_param1/1 -> wheel vel cntr/1(platform_dxdy_cntr_param)
  disable1/1 -> wheel vel cntr/2(disable)
  ena_w/1 -> wheel vel cntr/4(ena_w)
  dvarphi/1 -> wheel vel cntr/5(dvarphi)

== system ROPOD_4Wheel_Tdistkinb_cntr_modular_Code_GEN/Subsystem/Ropod kinematic parameters ==
  ropod_kinmodel_pv : Constant  Value=ropod_kinmodel_pv
  ropod_kin_param : Outport  VectorParamsAs1DForOutWhenUnconnected=off
  wires:
  ropod_kinmodel_pv/1 -> ropod_kin_param/1

== system ROPOD_4Wheel_Tdistkinb_cntr_modular_Code_GEN/Subsystem/Smart wheels conf1 ==
  Bus Creator : BusCreator  Inputs=8
  LPF_fhz_ddelta_meas : Constant  Value=LPF_fhz_ddelta_meas
  LPF_fhz_dvarphi_meas : Constant  Value=LPF_fhz_dvarphi_meas
  enable : Constant
  max_current : Constant  Value=max_sw_current
  pivot_offset_sw1 : Constant  Value=pivot_offs_sws(1)
  pivot_offset_sw2 : Constant  Value=pivot_offs_sws(2)
  pivot_offset_sw3 : Constant  Value=pivot_offs_sws(3)
  pivot_offset_sw4 : Constant  Value=pivot_offs_sws(4)
  sw_conf : Outport  VectorParamsAs1DForOutWhenUnconnected=off
  wires:
  enable/1 -> Bus Creator/1  "enable"
  Bus Creator/1 -> sw_conf/1
  max_current/1 -> Bus Creator/2  "max_current"
  pivot_offset_sw1/1 -> Bus Creator/3  "pivot_offs_sw1"
  pivot_offset_sw2/1 -> Bus Creator/4  "pivot_offs_sw2"
  pivot_offset_sw3/1 -> Bus Creator/5  "pivot_offs_sw3"
  pivot_offset_sw4/1 -> Bus Creator/6  "pivot_offs_sw4"
  LPF_fhz_dvarphi_meas/1 -> Bus Creator/7  "dvarphi_LPF_fhz"
  LPF_fhz_ddelta_meas/1 -> Bus Creator/8  "ddelta_LPF_fhz"

== system ROPOD_4Wheel_Tdistkinb_cntr_modular_Code_GEN/RopodTorqueDistribution/ROPOD 4SW/Initialization switch ==
  ropod_cntr_mode : Inport
  curr_setp : Inport  Port=2
  Constant1 : Constant  Value=SW_COM1_MODE_TORQUE
  Constant13 : Constant  Value=SW_COM1_MODE_TORQUE
  Constant5 : Constant  Value=SW_COM1_MODE_VELOCITY
  Index Vector : MultiPortSwitch  DataPortOrder=Zero-based contiguous  zeroidx=on
  Index Vector1 : MultiPortSwitch  DataPortOrder=Zero-based contiguous  zeroidx=on
  Movinf around SW axis center : Constant  Value=[2 -2 2 -2 2 -2 2 -2]
  zeros : Constant  Value=[0 0 0 0 0 0 0 0]
  SW_cntr_mode : Outport  VectorParamsAs1DForOutWhenUnconnected=off
  wheel_setp : Outport  Port=2  VectorParamsAs1DForOutWhenUnconnected=off
  wires:
  ropod_cntr_mode/1 -> Index Vector1/1, Index Vector/1
  Constant1/1 -> Index Vector/2
  zeros/1 -> Index Vector1/2
  Index Vector1/1 -> wheel_setp/1
  Index Vector/1 -> SW_cntr_mode/1
  Constant5/1 -> Index Vector/4
  Constant13/1 -> Index Vector/3
  Movinf around SW axis center/1 -> Index Vector1/4
  curr_setp/1 -> Index Vector1/3
